simulink model "legoway"  (R2020b)
settings: Solver=ode45  StartTime=0.0  StopTime=30  RelTol=1e-3
values from neighbouring files (symbols this model uses):
  cs = getHipsterSS()    [init.m]
  dpsi_0 = 0    [init.m]
  dx_0 = 0    [init.m]
  f_a_delay = [0;0]    [init.m]
  f_a_gain = [ 1 ; 1]    [init.m]
  f_a_offset = [ 0 ; 0]    [init.m]
  f_s_drift = [0;0;0]    [init.m]
  f_s_offset = [0;0;0]    [init.m]
  f_t = [fault_start;fault_stop]    [init.m]
  psi_0 = 0    [init.m]
  rC = [r0;r1;r2;r34]    [init.m]
  reg_d = c2d(reg_c,Ts)    [lqg_legoway.m]
  Ts = 2E-3    (= 0.002)    [init.m]
  x_0 = 0    [init.m]
  yuw = yu_window(ns,Ts)    [init.m]
libraries: simulink x7, dspstat3 x3, dspmathops x2
settings Model: PacingRate=0.110000  Creator=dirk  LastModifiedBy=dirk

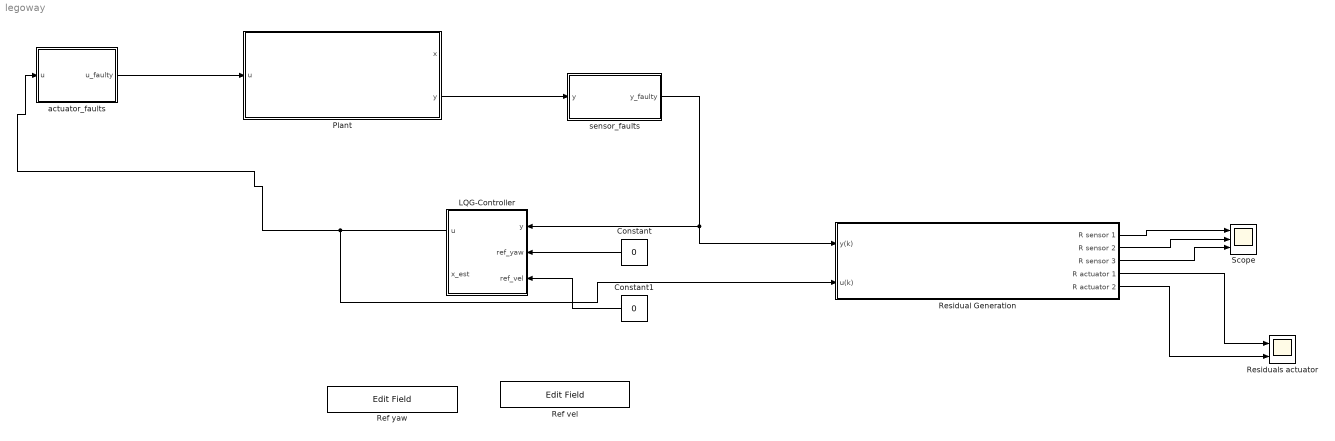
== system legoway ==
  Constant : Constant  Value=0
  Constant1 : Constant  Value=0
  LQG-Controller : Subsystem
  Plant : Subsystem
  Ref vel : EditField  LabelPosition=Hide  ShowInitialText=on  Alignment=Center
  Ref yaw : EditField  LabelPosition=Hide  ShowInitialText=on  Alignment=Center
  Residual Generation : Subsystem
  Residuals actuator : Scope  NumInputPorts=2
  Scope : Scope  NumInputPorts=3
  actuator_faults : Subsystem
  sensor_faults : Subsystem
  wires:
  sensor_faults/1(y_faulty) -> Residual Generation/1(y(k)), LQG-Controller/1(y)
  Constant/1 -> LQG-Controller/2(ref_yaw)
  Constant1/1 -> LQG-Controller/3(ref_vel)
  actuator_faults/1(u_faulty) -> Plant/1(u)
  Plant/2(y) -> sensor_faults/1(y)
  LQG-Controller/1(u) -> Residual Generation/2(u(k)), actuator_faults/1(u)
  Residual Generation/4(R actuator 1) -> Residuals actuator/1
  Residual Generation/5(R actuator 2) -> Residuals actuator/2
  Residual Generation/1(R sensor 1) -> Scope/1
  Residual Generation/2(R sensor 2) -> Scope/2
  Residual Generation/3(R sensor 3) -> Scope/3

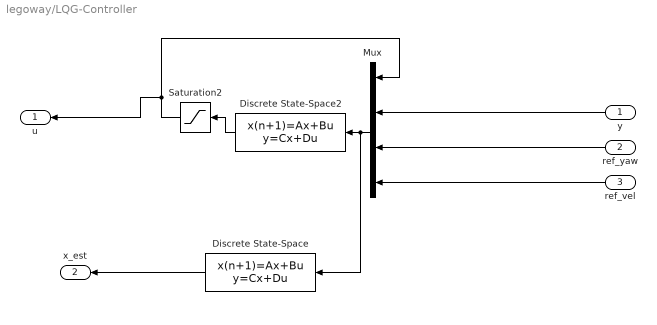
== system legoway/LQG-Controller ==
  y : Inport
  ref_yaw : Inport  Port=2
  ref_vel : Inport  Port=3
  Discrete State-Space : DiscreteStateSpace  A=reg_d.A  B=reg_d.B  C=diag(ones(1,8))  D=zeros(8,7)  SampleTime=Ts
  Discrete State-Space2 : DiscreteStateSpace  A=reg_d.A  B=reg_d.B  C=reg_d.C  D=reg_d.D  SampleTime=Ts
  Mux : Mux
  Saturation2 : Saturate  UpperLimit=8  LowerLimit=-8
  u : Outport
  x_est : Outport  Port=2
  wires:
  y/1 -> Mux/2
  ref_yaw/1 -> Mux/3
  Saturation2/1 -> u/1, Mux/1
  Discrete State-Space2/1 -> Saturation2/1
  ref_vel/1 -> Mux/4
  Mux/1 -> Discrete State-Space/1, Discrete State-Space2/1
  Discrete State-Space/1 -> x_est/1

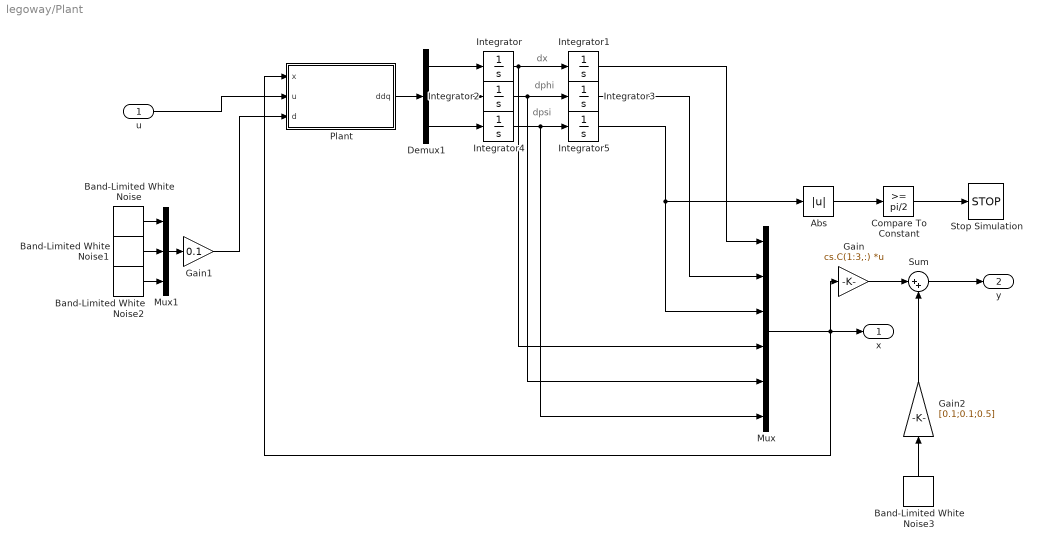
== system legoway/Plant ==
  note: dpsi
  note: dphi
  note: dx
  u : Inport
  Abs : Abs
  Band-Limited White Noise : simulink/Sources/Band-Limited White Noise  Cov=[0.01]  Ts=0.1  seed=[23341]
  Band-Limited White Noise1 : simulink/Sources/Band-Limited White Noise  Cov=[0.01]  Ts=0.1  seed=[32654]
  Band-Limited White Noise2 : simulink/Sources/Band-Limited White Noise  Cov=[0.01]  Ts=0.1  seed=[2341]
  Band-Limited White Noise3 : simulink/Sources/Band-Limited White Noise  Cov=[0.005]  Ts=0.01  seed=[23132]
  Compare To Constant : simulink/Logic and Bit Operations/Compare To Constant  relop=>=  const=pi/2  OutDataTypeStr=boolean
  Demux1 : Demux  Outputs=3
  Gain : Gain  Gain=cs.C(1:3,:)  Multiplication=Matrix(K*u)
  Gain1 : Gain  Gain=0.1
  Gain2 : Gain  Gain=[0.1;0.1;0.5]
  Integrator : Integrator  InitialCondition=dx_0
  Integrator1 : Integrator  InitialCondition=x_0
  Integrator2 : Integrator
  Integrator3 : Integrator
  Integrator4 : Integrator  InitialCondition=dpsi_0
  Integrator5 : Integrator  InitialCondition=psi_0  UpperSaturationLimit=pi/2  LowerSaturationLimit=-pi/2
  Mux : Mux  Inputs=6
  Mux1 : Mux  Inputs=3
  Plant : MATLAB Function  TreatAsAtomicUnit=on
  Stop Simulation : Stop
  Sum : Sum  Inputs=|++
  x : Outport
  y : Outport  Port=2
  wires:
  Abs/1 -> Compare To Constant/1
  Demux1/3 -> Integrator4/1
  Demux1/1 -> Integrator/1
  Plant/1(ddq) -> Demux1/1
  Integrator4/1 -> Mux/6, Integrator5/1
  Integrator2/1 -> Mux/5, Integrator3/1
  Demux1/2 -> Integrator2/1
  Integrator/1 -> Mux/4, Integrator1/1
  u/1 -> Plant/2(u)
  Integrator3/1 -> Mux/2
  Integrator1/1 -> Mux/1
  Integrator5/1 -> Mux/3, Abs/1
  Compare To Constant/1 -> Stop Simulation/1
  Mux/1 -> x/1, Gain/1, Plant/1(x)
  Sum/1 -> y/1
  Band-Limited White Noise/1 -> Mux1/1
  Band-Limited White Noise1/1 -> Mux1/2
  Band-Limited White Noise2/1 -> Mux1/3
  Mux1/1 -> Gain1/1
  Gain/1 -> Sum/1
  Gain1/1 -> Plant/3(d)
  Band-Limited White Noise3/1 -> Gain2/1
  Gain2/1 -> Sum/2

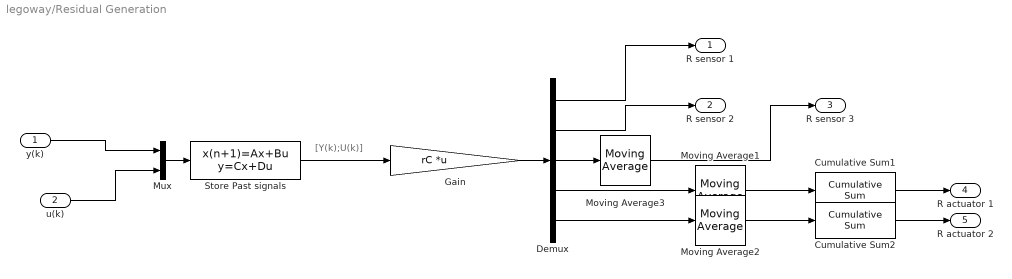
== system legoway/Residual Generation ==
  note: [Y(k);U(k)]
  y(k) : Inport
  u(k) : Inport  Port=2
  Cumulative Sum1 : dspmathops/Cumulative Sum  dim=Channels (running sum)  InputProcessing=Columns as channels (frame based)  reset_popup=None  roundingMode=Floor  overflowMode=off  outputDataTypeStr=Inherit: Same as accumulator  outputMin=[]  outputMax=[]  outputLastDataTypeStr=Inherit: Same as accumulator
  Cumulative Sum2 : dspmathops/Cumulative Sum  dim=Channels (running sum)  InputProcessing=Columns as channels (frame based)  reset_popup=None  roundingMode=Floor  overflowMode=off  outputDataTypeStr=Inherit: Same as accumulator  outputMin=[]  outputMax=[]  outputLastDataTypeStr=Inherit: Same as accumulator
  Demux : Demux  Outputs=5
  Gain : Gain  Gain=rC  Multiplication=Matrix(K*u)
  Moving Average1 : dspstat3/Moving Average  Method=Sliding window  ForgettingFactorPort=off  SpecifyWindowLength=on  WindowLength=10  ForgettingFactor=0.9  SimulateUsing=Code generation
  Moving Average2 : dspstat3/Moving Average  Method=Sliding window  ForgettingFactorPort=off  SpecifyWindowLength=on  WindowLength=10  ForgettingFactor=0.9  SimulateUsing=Code generation
  Moving Average3 : dspstat3/Moving Average  Method=Sliding window  ForgettingFactorPort=off  SpecifyWindowLength=on  WindowLength=10  ForgettingFactor=0.9  SimulateUsing=Code generation
  Mux : Mux  Inputs=2
  Store Past signals : DiscreteStateSpace  A=yuw.A  B=yuw.B  C=yuw.C  D=yuw.D  SampleTime=Ts
  R sensor 1 : Outport
  R sensor 2 : Outport  Port=2
  R sensor 3 : Outport  Port=3
  R actuator 1 : Outport  Port=4
  R actuator 2 : Outport  Port=5
  wires:
  Store Past signals/1 -> Gain/1
  Gain/1 -> Demux/1
  Demux/5 -> Moving Average2/1
  Mux/1 -> Store Past signals/1
  Demux/4 -> Moving Average1/1
  Moving Average2/1 -> Cumulative Sum2/1
  Demux/2 -> R sensor 2/1
  Moving Average1/1 -> Cumulative Sum1/1
  Cumulative Sum2/1 -> R actuator 2/1
  y(k)/1 -> Mux/1
  u(k)/1 -> Mux/2
  Demux/1 -> R sensor 1/1
  Demux/3 -> Moving Average3/1
  Cumulative Sum1/1 -> R actuator 1/1
  Moving Average3/1 -> R sensor 3/1

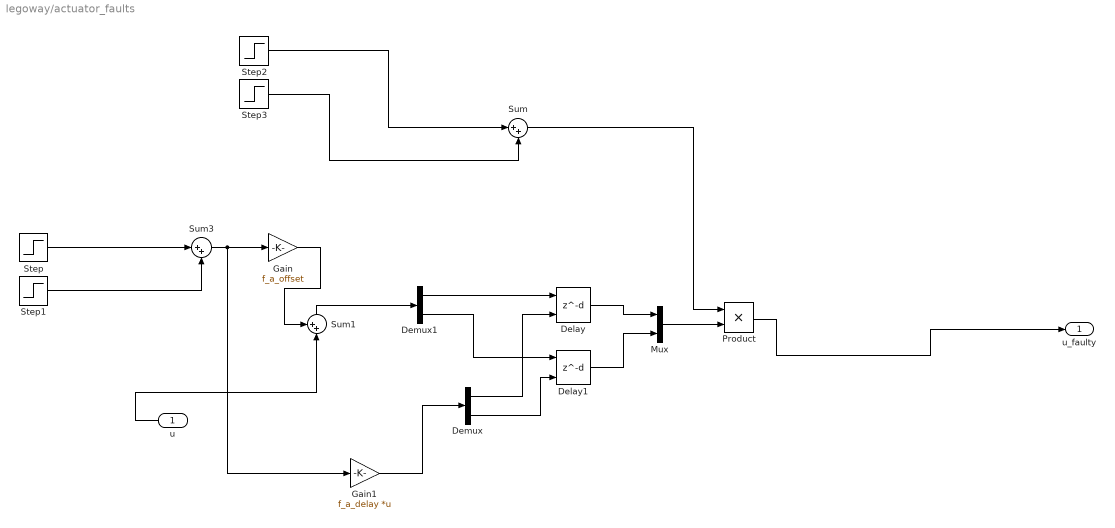
== system legoway/actuator_faults ==
  u : Inport
  Delay : Delay  DelayLengthSource=Input port  DelayLength=100  DelayLengthUpperLimit=1000  SampleTime=Ts
      settings: InputPortMap=u0,p1
  Delay1 : Delay  DelayLengthSource=Input port  DelayLength=100  DelayLengthUpperLimit=1000  SampleTime=Ts
      settings: InputPortMap=u0,p1
  Demux : Demux  Outputs=2
  Demux1 : Demux  Outputs=2
  Gain : Gain  Gain=f_a_offset
  Gain1 : Gain  Gain=f_a_delay  Multiplication=Matrix(K*u)
  Mux : Mux  Inputs=2
  Product : Product
  Step : Step  Time=f_t(1)  SampleTime=0
  Step1 : Step  Time=f_t(2)  After=-1  SampleTime=0
  Step2 : Step  Time=f_t(1)  Before=1  After=f_a_gain  SampleTime=0
  Step3 : Step  Time=f_t(2)  After=-f_a_gain + [1;1]  SampleTime=0
  Sum : Sum  Inputs=|++
  Sum1 : Sum  Inputs=++|
  Sum3 : Sum  Inputs=|++
  u_faulty : Outport
  wires:
  Sum1/1 -> Demux1/1
  Step/1 -> Sum3/1
  u/1 -> Sum1/2
  Product/1 -> u_faulty/1
  Step1/1 -> Sum3/2
  Delay/1 -> Mux/1
  Gain/1 -> Sum1/1
  Gain1/1 -> Demux/1
  Sum/1 -> Product/1
  Sum3/1 -> Gain1/1, Gain/1
  Demux1/1 -> Delay/1
  Demux1/2 -> Delay1/1
  Demux/1 -> Delay/2
  Demux/2 -> Delay1/2
  Mux/1 -> Product/2
  Delay1/1 -> Mux/2
  Step2/1 -> Sum/1
  Step3/1 -> Sum/2

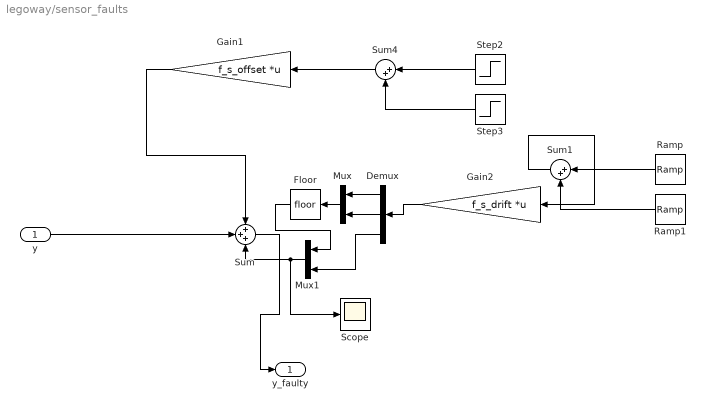
== system legoway/sensor_faults ==
  y : Inport
  Demux : Demux  Outputs=3
  Floor : Rounding
  Gain1 : Gain  Gain=f_s_offset  Multiplication=Matrix(K*u)
  Gain2 : Gain  Gain=f_s_drift  Multiplication=Matrix(K*u)
  Mux : Mux  Inputs=2
  Mux1 : Mux  Inputs=2
  Ramp : simulink/Sources/Ramp  slope=1  start=f_t(1)  InitialOutput=0
  Ramp1 : simulink/Sources/Ramp  slope=-1  start=f_t(2)  InitialOutput=0
  Scope : Scope
  Step2 : Step  Time=f_t(1)  SampleTime=0
  Step3 : Step  Time=f_t(2)  After=-1  SampleTime=0
  Sum : Sum  Inputs=+++
  Sum1 : Sum  Inputs=|++
  Sum4 : Sum  Inputs=|++
  y_faulty : Outport
  wires:
  Step3/1 -> Sum4/2
  Gain1/1 -> Sum/1
  Step2/1 -> Sum4/1
  y/1 -> Sum/2
  Sum4/1 -> Gain1/1
  Sum1/1 -> Gain2/1
  Ramp1/1 -> Sum1/2
  Ramp/1 -> Sum1/1
  Gain2/1 -> Demux/1
  Floor/1 -> Mux1/1
  Demux/2 -> Mux/2
  Demux/1 -> Mux/1
  Mux/1 -> Floor/1
  Demux/3 -> Mux1/2
  Mux1/1 -> Scope/1, Sum/3
  Sum/1 -> y_faulty/1

== matlab function legoway/Plant/Plant ==
  data: x input size=6; u input; d input size=3; ddq output size=3; const parameter
function ddq = legoway_nonlinear(x,u,d,const)

	% Load constants
	mw  = const.mw;     % wheel mass
	mb  = const.mb;     % body mass
	
	R   = const.R;      % wheel radius
	W   = const.W;      % half body width
	L   = const.L;      % length from wheel axle to center of mass
	Iw  = const.Iw;     % wheel moment of inertia
	Ij  = const.Ij;     % jaw moment of inertia
	Ip  = const.Ip;     % pitch moment of inertia
	Ixx = const.Ixx;
	Jm = const.Jm;      % tröghetsmoment för motorn
	g  = const.g;       % earth gravitation
	mc1 = const.mc1;    % motor constant 1 = Bm + Kt*Kb/Ra;
	mc2 = const.mc2;    % motor constant 2 = Kt/Ra;



	% Split state vector into inputs and q 
	% q = (x,phi,psi) 
	% dq = dq/dt
	% u = (V_left,V_right)
	q = x(1:3);
	dq = x(4:6);

	% Calculate the inertia matrix M(q)
	m11 = mb + 2*mw + 2*(Iw + Jm)/(R^2);
	m13 = mb*L*cos(q(3)) - 2 *(Jm/R);
	m22 = 2*(mw + (Iw + Jm)/(R^2))*W^2 + (Ixx + mb*L^2)*sin(q(3))^2 + Ij*cos(q(3))^2;
	m31 = m13;
	m33 = mb*L^2 + Ip + 2*Jm;

	M = [m11,0,m13 ; 0,m22,0 ; m31,0,m33];

	% Calculate the Coriolis matrix C(q,dq)
	c11 =(2/(R^2))*mc1;
	c13 = -(2/(R))*mc1-mb*L*sin(q(3))*dq(3);
	c22 = 2*((mb*L^2 + Ixx - Ij)*sin(q(3))*cos(q(3))*dq(3) + (W^2/(R^2))*mc1);
	c31 = -(2/(R))*mc1;
	c32 = -(mb*L^2 + Ixx - Ij)*sin(q(3))*cos(q(3))*dq(2) ;
	c33 = 2*mc1;

	C = [c11,0,c13 ; 0,c22,0 ; c31,c32,c33];

	% Calculate the gravity vector G(q)
	g3 = -mb*g*L*sin(q(3));
	G = [0;0;g3];

	% Calculate input tau 
	tau_u = [ mc2/R,mc2/R ; mc2*W/R,-mc2*W/R ; -mc2,-mc2];
	tau = tau_u*u;
    
   
	% The system dynamics are described by:
	% M(q)ddq + C(q,dq)dq + G(q) = tau
	% => ddq = M(q)\(-C(q,dq)dq - G(q) + tau) 
	
	ddq = M\(-C*dq - G + tau) + d;
end
